simulink model "online_fault_detection"  (R2015b)
settings: Solver=VariableStepAuto  StartTime=0.0  StopTime=10.0  RelTol=1e-3
values from neighbouring files (symbols this model uses):
  x2 = [VEa VEb VEc IEa IEb IEc V0 I0]    [final.m]    (also in final_online_classification.m = [va vb vc ia ib ic v0 i0]; final_online_detection.m = [va vb vc ia ib ic v0 i0]; final_online_detection1.m = [va vb vc ia ib ic v0 i0])
libraries: neural x105
(part 3 of 3)

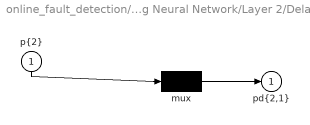
== system online_fault_detection/Function Fitting Neural Network/Layer 2/Delays 1 ==
  "p{2}" : Inport  PortDimensions=100
      mask Display: e = 0.06;c1 = [120 230 180]/255;c2 = ([120 230 180]+0)/(256+128);c3 = ([120 230 180]+128)/(256+128);patch([0 1 1 0],[0 0 1 1],c1);patch([0 1 1 1-e 1-e 0+e],[0 0 1 1-e 0+e 0+e],c2);patch([0 0 1 1-e 0+e 0+e],[0 1 1 1-e 1-e 0+e],c3);plot([0 1 1 0 0],[0 0 1 1 0]);
  mux : Mux  Inputs=1
      mask Display: e = 0.06;c1 = [120 150 230]/255;c2 = ([120 150 230]+0)/383;c3 = ([120 150 230]+128)/383;patch([0 1 1 0],[0 0 1 1],c1);patch([0 1 1 1-e 1-e 0+e],[0 0 1 1-e 0+e 0+e],c2);patch([0 0 1 1-e 0+e 0+e],[0 1 1 1-e 1-e 0+e],c3);plot([0 1 1 0 0],[0 0 1 1 0]);disp('Mux')
  "pd{2,1}" : Outport
      mask Display: e = 0.06;c1 = [120 230 180]/255;c2 = ([120 230 180]+0)/(256+128);c3 = ([120 230 180]+128)/(256+128);patch([0 1 1 0],[0 0 1 1],c1);patch([0 1 1 1-e 1-e 0+e],[0 0 1 1-e 0+e 0+e],c2);patch([0 0 1 1-e 0+e 0+e],[0 1 1 1-e 1-e 0+e],c3);plot([0 1 1 0 0],[0 0 1 1 0]);
  wires:
  "p{2}"/1 -> mux/1
  mux/1 -> "pd{2,1}"/1

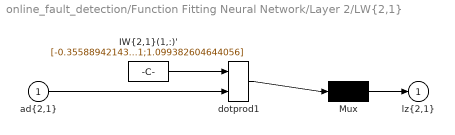
== system online_fault_detection/Function Fitting Neural Network/Layer 2/LW{2,1} ==
  "ad{2,1}" : Inport  PortDimensions=100
      mask Display: e = 0.06;c1 = [120 230 180]/255;c2 = ([120 230 180]+0)/(256+128);c3 = ([120 230 180]+128)/(256+128);patch([0 1 1 0],[0 0 1 1],c1);patch([0 1 1 1-e 1-e 0+e],[0 0 1 1-e 0+e 0+e],c2);patch([0 0 1 1-e 0+e 0+e],[0 1 1 1-e 1-e 0+e],c3);plot([0 1 1 0 0],[0 0 1 1 0]);
  "IW{2,1}(1,:)'" : Constant  Value=[-0.35588942143437874;-0.84047490541522174;0.28117081572097408;-0.055805910970702692;0.82575182173416639;-0.27308893368307396;0.091441189060658318;-0.67535130421029976;-0.22738360516471512;-0.54175581094379366;0.46697649219270099;0.87447205464764599;-0.13030801524175165;0.24534361829957455;-0.46855817160453361;0.005861820256575727;0.74706498886652284;0.36142049301196216;-0.41494435988645351;-0.32427433697854063;-0.17536906030982491;-0.226465586120698;-0.35650712192345263;0.07221666906874516;0.3310331426273822;-0.12785610691451735;-0.25962827853167614;-0.64528650176032754;-0.86325275841586213;-0.25043460856521033;-0.28730967042703348;0.30143034785596506;0.89703412733475785;0.77954297253695848;-0.011367007376782253;-0.41625048040493196;0.35736199826145204;0.27772602948728708;0.28642593036582015;0.56512380917259963;-0.68246059602324771;0.28408212794252102;-0.0051555347349197742;-0.57721537053026617;-0.73337809382210384;0.63178873078685083;-0.53007622234398288;-0.59245573662256978;0.31935903866522231;0.77734768366463391;0.13591999593399309;0.47384806128207857;-0.47461345428174428;0.89701664396277625;0.21012092167608226;0.4264541603046354;-0.96023697243451056;0.46735072469455374;0.6669253785725161;-0.69815848312466455;0.037319216708164862;-0.25280060711552921;0.11985761727910668;-0.15595326208157559;-0.035562860013550718;-0.56006041415409902;-0.34120365819021836;-0.92646692056420077;0.87855808668739621;0.31816340410540783;0.7646720351877907;-0.74776929441387474;0.62901488884508383;0.65323198017220097;0.11257129202265682;-0.0058924328925962699;-0.26898607476959652;0.54978202220090999;-0.4340340204564952;-0.88071743682097214;0.52152471438287207;0.27144367562149124;0.44991387781721137;0.10594216718858016;-0.11411017873002144;-0.030342420878532842;0.38388367176271071;-0.12901523065843443;0.81656850354020116;0.48947937679915715;0.5593301543826269;-0.0034070407578448555;0.12310799247549131;0.89491206856358574;-0.091609108455466867;-0.80421790632745926;0.68571713932027367;0.39338891586487384;-0.41257873414976481;1.099382604644056]
      mask Display: e = 0.06;c1 = [120 150 230]/255;c2 = ([120 150 230]+0)/383;c3 = ([120 150 230]+128)/383;patch([0 1 1 0],[0 0 1 1],c1);patch([0 1 1 1-e 1-e 0+e],[0 0 1 1-e 0+e 0+e],c2);patch([0 0 1 1-e 0+e 0+e],[0 1 1 1-e 1-e 0+e],c3);plot([0 1 1 0 0],[0 0 1 1 0]);disp('weights');
  Mux : Mux  Inputs=1
      mask Display: e = 0.06;c1 = [120 150 230]/255;c2 = ([120 150 230]+0)/383;c3 = ([120 150 230]+128)/383;patch([0 1 1 0],[0 0 1 1],c1);patch([0 1 1 1-e 1-e 0+e],[0 0 1 1-e 0+e 0+e],c2);patch([0 0 1 1-e 0+e 0+e],[0 1 1 1-e 1-e 0+e],c3);plot([0 1 1 0 0],[0 0 1 1 0]);disp('Mux');
  dotprod1 : neural/Weight Functions/dotprod
  "lz{2,1}" : Outport
      mask Display: e = 0.06;c1 = [120 230 180]/255;c2 = ([120 230 180]+0)/(256+128);c3 = ([120 230 180]+128)/(256+128);patch([0 1 1 0],[0 0 1 1],c1);patch([0 1 1 1-e 1-e 0+e],[0 0 1 1-e 0+e 0+e],c2);patch([0 0 1 1-e 0+e 0+e],[0 1 1 1-e 1-e 0+e],c3);plot([0 1 1 0 0],[0 0 1 1 0]);
  wires:
  "IW{2,1}(1,:)'"/1 -> dotprod1/1
  "ad{2,1}"/1 -> dotprod1/2
  dotprod1/1 -> Mux/1
  Mux/1 -> "lz{2,1}"/1
